simulink model "Y6MultirotorOpenLoopModelSimulation"  (R2019b)
settings: Solver=ode45  StartTime=0.0  StopTime=10  RelTol=1e-3  EnableMultiTasking=on
undefined symbols (not defined in the file or in its folder): Dxx, Dyy, Dzz, Ixx, Iyy, Izz, Ktau, Kthrust, Ku, Kw, L1, L2, L3, M, Mtau, U_e
settings Model: Creator=bjones  LastModifiedBy=alexd
settings DataIOCC: LimitDataPoints=on  SaveFormat=Array  SignalLoggingSaveFormat=ModelDataLogs  ReturnWorkspaceOutputs=off
settings OptimizationCC: ExpressionDepthLimit=2147483647  LifeSpan=inf
settings DebuggingCC: UnderspecifiedInitializationDetection=Classic  MergeDetectMultiDrivingBlocksExec=none  FcnCallInpInsideContextMsg=warning  StateNameClashWarn=warning  SFUnexpectedBacktrackingDiag=warning  SFNoUnconditionalDefaultTransitionDiag=warning  SFExecutionAtInitializationDiag=none  ArithmeticOperatorsInVariantConditions=warning
settings HardwareCC: ProdBitPerPointer=32  ProdBitPerSizeT=32  ProdBitPerPtrDiffT=32  ProdLargestAtomicFloat=None  ProdIntDivRoundTo=Undefined  ProdEndianess=Unspecified  ProdWordSize=32  ProdHWDeviceType=32-bit Generic
settings ModelReferenceCC: PropagateSignalLabelsOutOfModel=off
settings SFSimCC: SimUseLocalCustomCode=off  CustomCodeUndefinedFunction=UseInterfaceOnly
settings RTWCC: RTWUseLocalCustomCode=off
settings CodeAppCC: StateflowObjectComments=on
settings GRTTargetCC: TargetLangStandard=C89/C90 (ANSI)  GeneratePreprocessorConditionals=Disable all  CombineOutputUpdateFcns=off  GRTInterface=on
settings ConfigComp: CovMetricSettings=dw  CovHtmlReporting=on  CovSaveCumulativeToWorkspaceVar=on  CovSaveSingleToWorkspaceVar=on  CovExternalEMLEnable=off  CovSFcnEnable=off

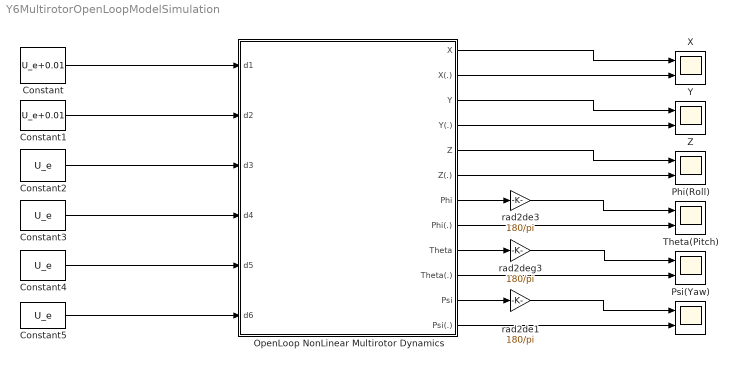
== system Y6MultirotorOpenLoopModelSimulation ==
  Constant : Constant  Value=U_e+0.01
  Constant1 : Constant  Value=U_e+0.01
  Constant{2..5} (4 alike) : Constant  Value=U_e
  OpenLoop NonLinear Multirotor Dynamics : Subsystem
  Phi(Roll) : Scope  NumInputPorts=2
  Psi(Yaw) : Scope  NumInputPorts=2
  Theta(Pitch) : Scope  NumInputPorts=2
  X : Scope  NumInputPorts=2
  Y : Scope  NumInputPorts=2
  Z : Scope  NumInputPorts=2
  rad2de1 : Gain  Gain=180/pi  SaturateOnIntegerOverflow=on  OutDataTypeStr=Inherit: Same as input  ParamDataTypeStr=Inherit: Same as input
  rad2de3 : Gain  Gain=180/pi  SaturateOnIntegerOverflow=on  OutDataTypeStr=Inherit: Same as input  ParamDataTypeStr=Inherit: Same as input
  rad2deg3 : Gain  Gain=180/pi  SaturateOnIntegerOverflow=on  OutDataTypeStr=Inherit: Same as input  ParamDataTypeStr=Inherit: Same as input
  wires:
  OpenLoop NonLinear Multirotor Dynamics/5(Z) -> Z/1
  OpenLoop NonLinear Multirotor Dynamics/1(X) -> X/1
  rad2deg3/1 -> Theta(Pitch)/1
  Constant/1 -> OpenLoop NonLinear Multirotor Dynamics/1(d1)
  Constant1/1 -> OpenLoop NonLinear Multirotor Dynamics/2(d2)
  OpenLoop NonLinear Multirotor Dynamics/3(Y) -> Y/1
  rad2de1/1 -> Psi(Yaw)/1
  rad2de3/1 -> Phi(Roll)/1
  Constant2/1 -> OpenLoop NonLinear Multirotor Dynamics/3(d3)
  Constant3/1 -> OpenLoop NonLinear Multirotor Dynamics/4(d4)
  Constant4/1 -> OpenLoop NonLinear Multirotor Dynamics/5(d5)
  Constant5/1 -> OpenLoop NonLinear Multirotor Dynamics/6(d6)
  OpenLoop NonLinear Multirotor Dynamics/7(Phi) -> rad2de3/1
  OpenLoop NonLinear Multirotor Dynamics/9(Theta) -> rad2deg3/1
  OpenLoop NonLinear Multirotor Dynamics/11(Psi) -> rad2de1/1
  OpenLoop NonLinear Multirotor Dynamics/12(Psi(.)) -> Psi(Yaw)/2
  OpenLoop NonLinear Multirotor Dynamics/10(Theta(.)) -> Theta(Pitch)/2
  OpenLoop NonLinear Multirotor Dynamics/8(Phi(.)) -> Phi(Roll)/2
  OpenLoop NonLinear Multirotor Dynamics/6(Z(.)) -> Z/2
  OpenLoop NonLinear Multirotor Dynamics/4(Y(.)) -> Y/2
  OpenLoop NonLinear Multirotor Dynamics/2(X(.)) -> X/2

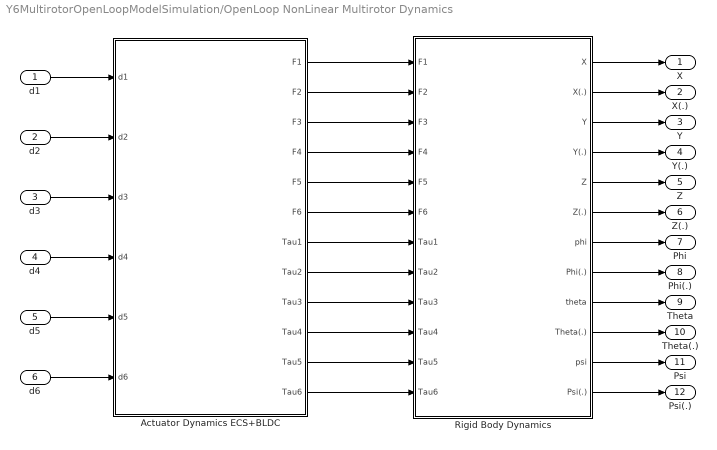
== system Y6MultirotorOpenLoopModelSimulation/OpenLoop NonLinear Multirotor Dynamics ==
  d1 : Inport
  d2 : Inport  Port=2
  d3 : Inport  Port=3
  d4 : Inport  Port=4
  d5 : Inport  Port=5
  d6 : Inport  Port=6
  Actuator Dynamics ECS+BLDC : Subsystem
  Rigid Body Dynamics : Subsystem
  X : Outport  VectorParamsAs1DForOutWhenUnconnected=off
  X(.) : Outport  Port=2  VectorParamsAs1DForOutWhenUnconnected=off
  Y : Outport  Port=3  VectorParamsAs1DForOutWhenUnconnected=off
  Y(.) : Outport  Port=4  VectorParamsAs1DForOutWhenUnconnected=off
  Z : Outport  Port=5  VectorParamsAs1DForOutWhenUnconnected=off
  Z(.) : Outport  Port=6  VectorParamsAs1DForOutWhenUnconnected=off
  Phi : Outport  Port=7  VectorParamsAs1DForOutWhenUnconnected=off
  Phi(.) : Outport  Port=8  VectorParamsAs1DForOutWhenUnconnected=off
  Theta : Outport  Port=9  VectorParamsAs1DForOutWhenUnconnected=off
  Theta(.) : Outport  Port=10  VectorParamsAs1DForOutWhenUnconnected=off
  Psi : Outport  Port=11  VectorParamsAs1DForOutWhenUnconnected=off
  Psi(.) : Outport  Port=12  VectorParamsAs1DForOutWhenUnconnected=off
  wires:
  Rigid Body Dynamics/7(phi) -> Phi/1
  Rigid Body Dynamics/8(Phi(.)) -> Phi(.)/1
  Rigid Body Dynamics/9(theta) -> Theta/1
  Rigid Body Dynamics/10(Theta(.)) -> Theta(.)/1
  Rigid Body Dynamics/11(psi) -> Psi/1
  Rigid Body Dynamics/12(Psi(.)) -> Psi(.)/1
  d1/1 -> Actuator Dynamics ECS+BLDC/1(d1)
  d2/1 -> Actuator Dynamics ECS+BLDC/2(d2)
  d3/1 -> Actuator Dynamics ECS+BLDC/3(d3)
  d4/1 -> Actuator Dynamics ECS+BLDC/4(d4)
  d5/1 -> Actuator Dynamics ECS+BLDC/5(d5)
  d6/1 -> Actuator Dynamics ECS+BLDC/6(d6)
  Actuator Dynamics ECS+BLDC/12(Tau6) -> Rigid Body Dynamics/12(Tau6)
  Actuator Dynamics ECS+BLDC/11(Tau5) -> Rigid Body Dynamics/11(Tau5)
  Actuator Dynamics ECS+BLDC/10(Tau4) -> Rigid Body Dynamics/10(Tau4)
  Actuator Dynamics ECS+BLDC/9(Tau3) -> Rigid Body Dynamics/9(Tau3)
  Actuator Dynamics ECS+BLDC/8(Tau2) -> Rigid Body Dynamics/8(Tau2)
  Actuator Dynamics ECS+BLDC/7(Tau1) -> Rigid Body Dynamics/7(Tau1)
  Actuator Dynamics ECS+BLDC/6(F6) -> Rigid Body Dynamics/6(F6)
  Actuator Dynamics ECS+BLDC/5(F5) -> Rigid Body Dynamics/5(F5)
  Actuator Dynamics ECS+BLDC/4(F4) -> Rigid Body Dynamics/4(F4)
  Actuator Dynamics ECS+BLDC/3(F3) -> Rigid Body Dynamics/3(F3)
  Actuator Dynamics ECS+BLDC/2(F2) -> Rigid Body Dynamics/2(F2)
  Actuator Dynamics ECS+BLDC/1(F1) -> Rigid Body Dynamics/1(F1)
  Rigid Body Dynamics/6(Z(.)) -> Z(.)/1
  Rigid Body Dynamics/5(Z) -> Z/1
  Rigid Body Dynamics/4(Y(.)) -> Y(.)/1
  Rigid Body Dynamics/3(Y) -> Y/1
  Rigid Body Dynamics/2(X(.)) -> X(.)/1
  Rigid Body Dynamics/1(X) -> X/1

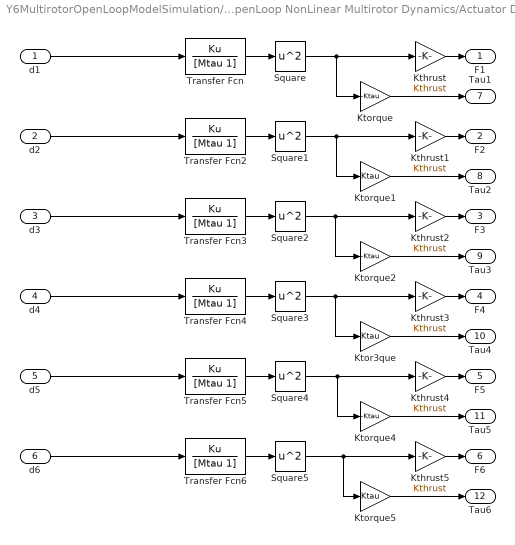
== system Y6MultirotorOpenLoopModelSimulation/OpenLoop NonLinear Multirotor Dynamics/Actuator Dynamics ECS+BLDC ==
  d1 : Inport
  d2 : Inport  Port=2
  d3 : Inport  Port=3
  d4 : Inport  Port=4
  d5 : Inport  Port=5
  d6 : Inport  Port=6
  Kthrust{,1..5} (6 alike) : Gain  Gain=Kthrust
  Ktor3que : Gain  Gain=Ktau
  Ktorque : Gain  Gain=-Ktau
  Ktorque1 : Gain  Gain=Ktau
  Ktorque2 : Gain  Gain=-Ktau
  Ktorque4 : Gain  Gain=-Ktau
  Ktorque5 : Gain  Gain=Ktau
  Square{,1..5} (6 alike) : Math  Operator=square  SignedPower=off  SaturateOnIntegerOverflow=on
  Transfer Fcn{,2..6} (6 alike) : TransferFcn  Numerator=Ku  Denominator=[Mtau 1]
  F1 : Outport  VectorParamsAs1DForOutWhenUnconnected=off
  F2 : Outport  Port=2  VectorParamsAs1DForOutWhenUnconnected=off
  F3 : Outport  Port=3  VectorParamsAs1DForOutWhenUnconnected=off
  F4 : Outport  Port=4  VectorParamsAs1DForOutWhenUnconnected=off
  F5 : Outport  Port=5  VectorParamsAs1DForOutWhenUnconnected=off
  F6 : Outport  Port=6  VectorParamsAs1DForOutWhenUnconnected=off
  Tau1 : Outport  Port=7  VectorParamsAs1DForOutWhenUnconnected=off
  Tau2 : Outport  Port=8  VectorParamsAs1DForOutWhenUnconnected=off
  Tau3 : Outport  Port=9  VectorParamsAs1DForOutWhenUnconnected=off
  Tau4 : Outport  Port=10  VectorParamsAs1DForOutWhenUnconnected=off
  Tau5 : Outport  Port=11  VectorParamsAs1DForOutWhenUnconnected=off
  Tau6 : Outport  Port=12  VectorParamsAs1DForOutWhenUnconnected=off
  wires:
  Transfer Fcn/1 -> Square/1
  d1/1 -> Transfer Fcn/1
  d2/1 -> Transfer Fcn2/1
  d3/1 -> Transfer Fcn3/1
  d4/1 -> Transfer Fcn4/1
  d5/1 -> Transfer Fcn5/1
  d6/1 -> Transfer Fcn6/1
  Transfer Fcn2/1 -> Square1/1
  Transfer Fcn3/1 -> Square2/1
  Transfer Fcn4/1 -> Square3/1
  Transfer Fcn5/1 -> Square4/1
  Transfer Fcn6/1 -> Square5/1
  Ktorque/1 -> Tau1/1
  Ktorque1/1 -> Tau2/1
  Ktorque2/1 -> Tau3/1
  Ktor3que/1 -> Tau4/1
  Ktorque4/1 -> Tau5/1
  Ktorque5/1 -> Tau6/1
  Kthrust/1 -> F1/1
  Kthrust1/1 -> F2/1
  Kthrust2/1 -> F3/1
  Kthrust3/1 -> F4/1
  Kthrust4/1 -> F5/1
  Kthrust5/1 -> F6/1
  Square/1 -> Kthrust/1, Ktorque/1
  Square1/1 -> Kthrust1/1, Ktorque1/1
  Square2/1 -> Kthrust2/1, Ktorque2/1
  Square3/1 -> Kthrust3/1, Ktor3que/1
  Square4/1 -> Kthrust4/1, Ktorque4/1
  Square5/1 -> Kthrust5/1, Ktorque5/1

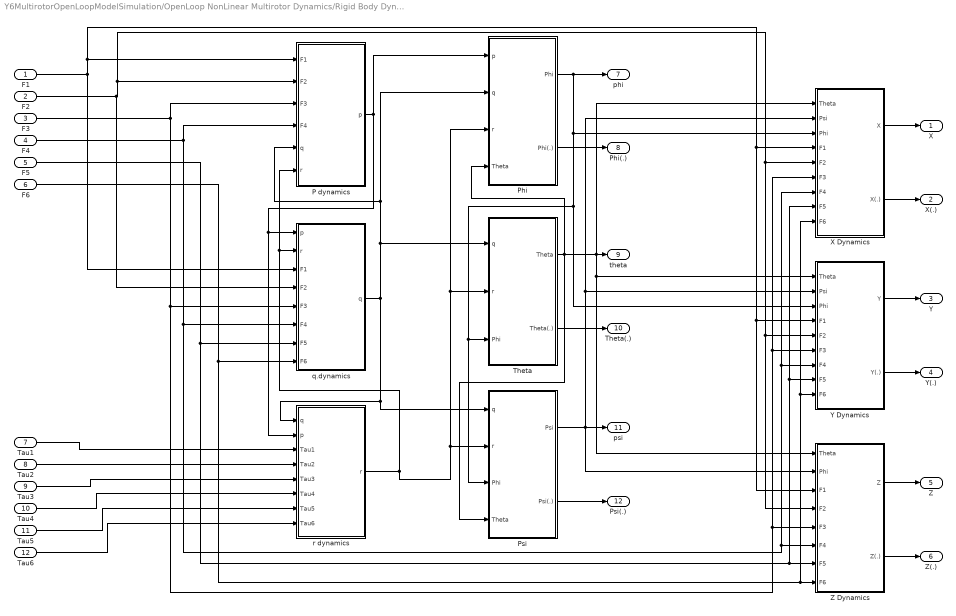
== system Y6MultirotorOpenLoopModelSimulation/OpenLoop NonLinear Multirotor Dynamics/Rigid Body Dynamics ==
  F1 : Inport
  F2 : Inport  Port=2
  F3 : Inport  Port=3
  F4 : Inport  Port=4
  F5 : Inport  Port=5
  F6 : Inport  Port=6
  Tau1 : Inport  Port=7
  Tau2 : Inport  Port=8
  Tau3 : Inport  Port=9
  Tau4 : Inport  Port=10
  Tau5 : Inport  Port=11
  Tau6 : Inport  Port=12
  P dynamics : Subsystem
  Phi : Subsystem
  Psi : Subsystem
  Theta : Subsystem
  X Dynamics : Subsystem
  Y Dynamics : Subsystem
  Z Dynamics : Subsystem
  q.dynamics : Subsystem
  r dynamics : Subsystem
  X : Outport  VectorParamsAs1DForOutWhenUnconnected=off
  X(.) : Outport  Port=2  VectorParamsAs1DForOutWhenUnconnected=off
  Y : Outport  Port=3  VectorParamsAs1DForOutWhenUnconnected=off
  Y(.) : Outport  Port=4  VectorParamsAs1DForOutWhenUnconnected=off
  Z : Outport  Port=5  VectorParamsAs1DForOutWhenUnconnected=off
  Z(.) : Outport  Port=6  VectorParamsAs1DForOutWhenUnconnected=off
  phi : Outport  Port=7  VectorParamsAs1DForOutWhenUnconnected=off
  Phi(.) : Outport  Port=8  VectorParamsAs1DForOutWhenUnconnected=off
  theta : Outport  Port=9  VectorParamsAs1DForOutWhenUnconnected=off
  Theta(.) : Outport  Port=10  VectorParamsAs1DForOutWhenUnconnected=off
  psi : Outport  Port=11  VectorParamsAs1DForOutWhenUnconnected=off
  Psi(.) : Outport  Port=12  VectorParamsAs1DForOutWhenUnconnected=off
  wires:
  Tau2/1 -> r dynamics/4(Tau2)
  Tau3/1 -> r dynamics/5(Tau3)
  Tau4/1 -> r dynamics/6(Tau4)
  Tau5/1 -> r dynamics/7(Tau5)
  Tau6/1 -> r dynamics/8(Tau6)
  F2/1 -> q.dynamics/4("F2 "), X Dynamics/5("F2 "), Z Dynamics/4("F2 "), Y Dynamics/5("F2 "), P dynamics/2(F2)
  F3/1 -> q.dynamics/5("F3 "), X Dynamics/6("F3 "), Y Dynamics/6("F3 "), Z Dynamics/5("F3 "), P dynamics/3(F3)
  F4/1 -> P dynamics/4(F4), q.dynamics/6("F4 "), X Dynamics/7("F4 "), Y Dynamics/7("F4 "), Z Dynamics/6("F4 ")
  Tau1/1 -> r dynamics/3(Tau1)
  r dynamics/1(r) -> Phi/3(r), Theta/2(r), Psi/2(r), P dynamics/6(r), q.dynamics/2(r)
  F1/1 -> Z Dynamics/3("F1 "), Y Dynamics/4("F1 "), X Dynamics/4("F1 "), P dynamics/1(F1), q.dynamics/3("F1 ")
  F5/1 -> q.dynamics/7("F5 "), Y Dynamics/8("F5 "), X Dynamics/8("F5 "), Z Dynamics/7("F5 ")
  F6/1 -> Y Dynamics/9(F6), X Dynamics/9(F6), Z Dynamics/8(F6), q.dynamics/8(F6)
  Z Dynamics/1(Z) -> Z/1
  Z Dynamics/2(Z(.)) -> Z(.)/1
  Y Dynamics/2(Y(.)) -> Y(.)/1
  Y Dynamics/1(Y) -> Y/1
  X Dynamics/2(X(.)) -> X(.)/1
  X Dynamics/1(X) -> X/1
  Phi/1(Phi) -> phi/1, X Dynamics/3(Phi), Y Dynamics/3(Phi), Theta/3(Phi), Psi/3(Phi)
  Theta/1(Theta) -> X Dynamics/1(Theta), theta/1, Y Dynamics/1(Theta), Z Dynamics/1(Theta), Phi/4(Theta), Psi/4(Theta)
  Theta/2(Theta(.)) -> Theta(.)/1
  Phi/2(Phi(.)) -> Phi(.)/1
  Psi/1(Psi) -> Z Dynamics/2(Phi), psi/1, X Dynamics/2(Psi), Y Dynamics/2(Psi)
  Psi/2(Psi(.)) -> Psi(.)/1
  q.dynamics/1(q) -> r dynamics/1(q), Psi/1(q), Theta/1(q), Phi/2(q), P dynamics/5(q)
  P dynamics/1(p) -> Phi/1(p), q.dynamics/1(p), r dynamics/2(p)

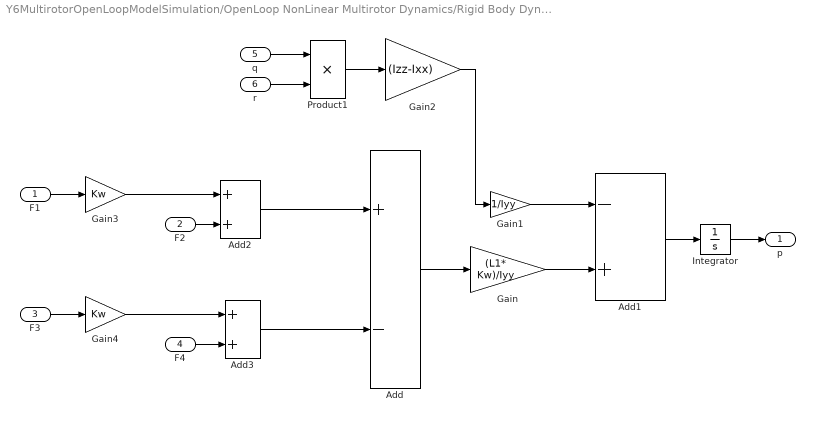
== system Y6MultirotorOpenLoopModelSimulation/OpenLoop NonLinear Multirotor Dynamics/Rigid Body Dynamics/P dynamics ==
  F1 : Inport
  F2 : Inport  Port=2
  F3 : Inport  Port=3
  F4 : Inport  Port=4
  q : Inport  Port=5
  r : Inport  Port=6
  Add : Sum  Inputs=+-
  Add1 : Sum  Inputs=-+
  Add2 : Sum
  Add3 : Sum
  Gain : Gain  Gain=(L1* Kw)/Iyy
  Gain1 : Gain  Gain=1/Iyy
  Gain2 : Gain  Gain=(Izz-Ixx)
  Gain3 : Gain  Gain=Kw
  Gain4 : Gain  Gain=Kw
  Integrator : Integrator
  Product1 : Product
  p : Outport  VectorParamsAs1DForOutWhenUnconnected=off
  wires:
  Product1/1 -> Gain2/1
  Add1/1 -> Integrator/1
  Gain1/1 -> Add1/1
  Add/1 -> Gain/1
  Gain2/1 -> Gain1/1
  Gain/1 -> Add1/2
  F4/1 -> Add3/2
  F3/1 -> Gain4/1
  Add2/1 -> Add/1
  Add3/1 -> Add/2
  Integrator/1 -> p/1
  r/1 -> Product1/2
  q/1 -> Product1/1
  F2/1 -> Add2/2
  F1/1 -> Gain3/1
  Gain3/1 -> Add2/1
  Gain4/1 -> Add3/1

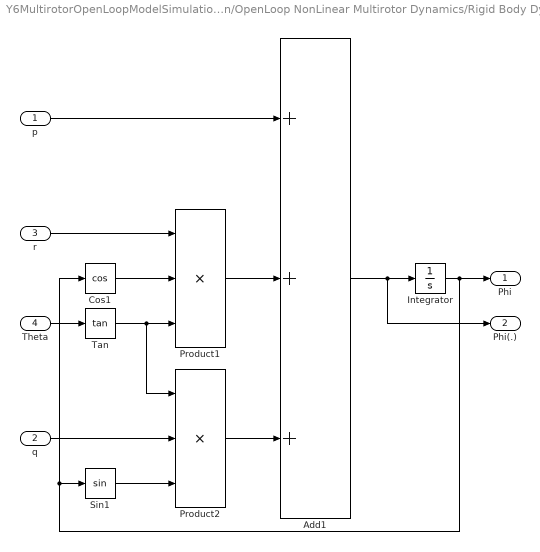
== system Y6MultirotorOpenLoopModelSimulation/OpenLoop NonLinear Multirotor Dynamics/Rigid Body Dynamics/Phi ==
  p : Inport
  q : Inport  Port=2
  r : Inport  Port=3
  Theta : Inport  Port=4
  Add1 : Sum  Inputs=+++
  Cos1 : Trigonometry  Operator=cos
  Integrator : Integrator
  Product1 : Product  Inputs=3
  Product2 : Product  Inputs=3
  Sin1 : Trigonometry
  Tan : Trigonometry  Operator=tan
  Phi : Outport  VectorParamsAs1DForOutWhenUnconnected=off
  Phi(.) : Outport  Port=2  VectorParamsAs1DForOutWhenUnconnected=off
  wires:
  p/1 -> Add1/1
  Theta/1 -> Tan/1
  Tan/1 -> Product2/1, Product1/3
  r/1 -> Product1/1
  Cos1/1 -> Product1/2
  Sin1/1 -> Product2/3
  q/1 -> Product2/2
  Product1/1 -> Add1/2
  Product2/1 -> Add1/3
  Add1/1 -> Phi(.)/1, Integrator/1
  Integrator/1 -> Cos1/1, Sin1/1, Phi/1

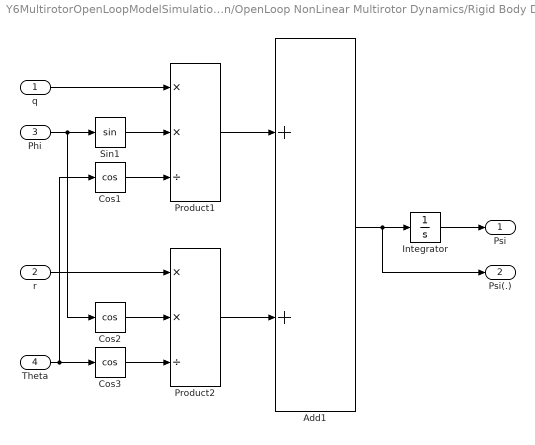
== system Y6MultirotorOpenLoopModelSimulation/OpenLoop NonLinear Multirotor Dynamics/Rigid Body Dynamics/Psi ==
  q : Inport
  r : Inport  Port=2
  Phi : Inport  Port=3
  Theta : Inport  Port=4
  Add1 : Sum
  Cos1 : Trigonometry  Operator=cos
  Cos2 : Trigonometry  Operator=cos
  Cos3 : Trigonometry  Operator=cos
  Integrator : Integrator
  Product1 : Product  Inputs=**/
  Product2 : Product  Inputs=**/
  Sin1 : Trigonometry
  Psi : Outport  VectorParamsAs1DForOutWhenUnconnected=off
  Psi(.) : Outport  Port=2  VectorParamsAs1DForOutWhenUnconnected=off
  wires:
  Add1/1 -> Integrator/1, Psi(.)/1
  Integrator/1 -> Psi/1
  Product1/1 -> Add1/1
  Product2/1 -> Add1/2
  Phi/1 -> Sin1/1, Cos2/1
  r/1 -> Product2/1
  q/1 -> Product1/1
  Cos2/1 -> Product2/2
  Cos3/1 -> Product2/3
  Theta/1 -> Cos1/1, Cos3/1
  Cos1/1 -> Product1/3
  Sin1/1 -> Product1/2

== system Y6MultirotorOpenLoopModelSimulation/OpenLoop NonLinear Multirotor Dynamics/Rigid Body Dynamics/Theta ==
  q : Inport
  r : Inport  Port=2
  Phi : Inport  Port=3
  Add1 : Sum  Inputs=+-
  Cos1 : Trigonometry  Operator=cos
  Integrator : Integrator
  Product1 : Product
  Product2 : Product
  Sin1 : Trigonometry
  Theta : Outport  VectorParamsAs1DForOutWhenUnconnected=off
  Theta(.) : Outport  Port=2  VectorParamsAs1DForOutWhenUnconnected=off
  wires:
  Cos1/1 -> Product1/2
  Add1/1 -> Integrator/1, Theta(.)/1
  Integrator/1 -> Theta/1
  Product1/1 -> Add1/1
  Product2/1 -> Add1/2
  Phi/1 -> Sin1/1, Cos1/1
  Sin1/1 -> Product2/2
  r/1 -> Product2/1
  q/1 -> Product1/1

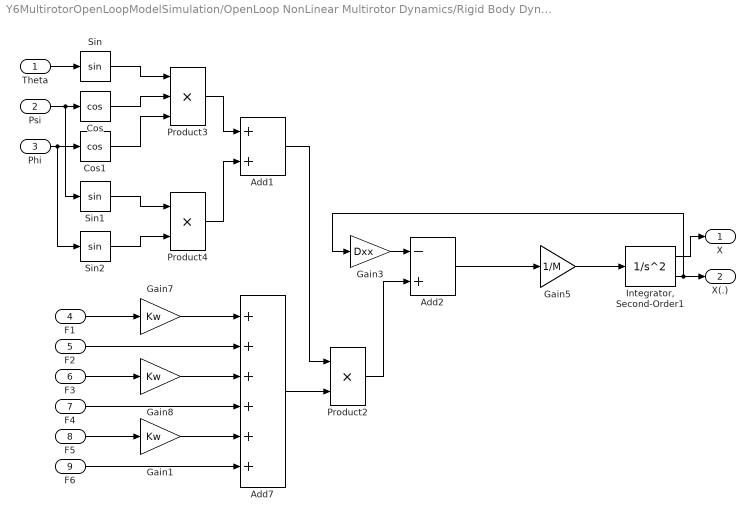
== system Y6MultirotorOpenLoopModelSimulation/OpenLoop NonLinear Multirotor Dynamics/Rigid Body Dynamics/X Dynamics ==
  Theta : Inport
  Psi : Inport  Port=2
  Phi : Inport  Port=3
  "F1 " : Inport  Port=4
  "F2 " : Inport  Port=5
  "F3 " : Inport  Port=6
  "F4 " : Inport  Port=7
  "F5 " : Inport  Port=8
  F6 : Inport  Port=9
  Add1 : Sum
  Add2 : Sum  Inputs=-+
  Add7 : Sum  Inputs=++++++
  Cos : Trigonometry  Operator=cos
  Cos1 : Trigonometry  Operator=cos
  Gain1 : Gain  Gain=Kw
  Gain3 : Gain  Gain=Dxx
  Gain5 : Gain  Gain=1/M
  Gain7 : Gain  Gain=Kw
  Gain8 : Gain  Gain=Kw
  "Integrator, Second-Order1" : SecondOrderIntegrator
  Product2 : Product
  Product3 : Product  Inputs=3
  Product4 : Product
  Sin : Trigonometry
  Sin1 : Trigonometry
  Sin2 : Trigonometry
  X : Outport  VectorParamsAs1DForOutWhenUnconnected=off
  X(.) : Outport  Port=2  VectorParamsAs1DForOutWhenUnconnected=off
  wires:
  "F4 "/1 -> Add7/4
  "F2 "/1 -> Add7/2
  "Integrator, Second-Order1"/2 -> X(.)/1, Gain3/1
  "F1 "/1 -> Gain7/1
  F6/1 -> Add7/6
  "F5 "/1 -> Gain1/1
  "F3 "/1 -> Gain8/1
  "Integrator, Second-Order1"/1 -> X/1
  Gain7/1 -> Add7/1
  Gain8/1 -> Add7/3
  Gain1/1 -> Add7/5
  Add7/1 -> Product2/2
  Theta/1 -> Sin/1
  Psi/1 -> Sin1/1, Cos/1
  Phi/1 -> Sin2/1, Cos1/1
  Sin/1 -> Product3/1
  Cos/1 -> Product3/2
  Cos1/1 -> Product3/3
  Product3/1 -> Add1/1
  Sin1/1 -> Product4/1
  Sin2/1 -> Product4/2
  Product4/1 -> Add1/2
  Add1/1 -> Product2/1
  Product2/1 -> Add2/2
  Add2/1 -> Gain5/1
  Gain3/1 -> Add2/1
  Gain5/1 -> "Integrator, Second-Order1"/1

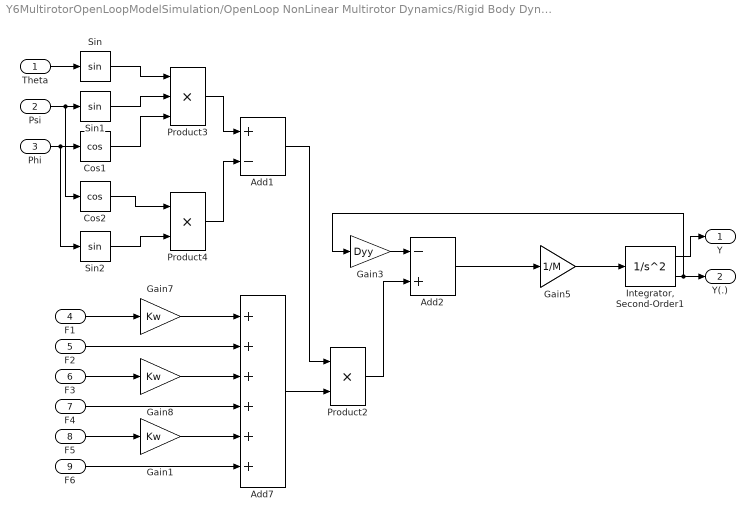
== system Y6MultirotorOpenLoopModelSimulation/OpenLoop NonLinear Multirotor Dynamics/Rigid Body Dynamics/Y Dynamics ==
  Theta : Inport
  Psi : Inport  Port=2
  Phi : Inport  Port=3
  "F1 " : Inport  Port=4
  "F2 " : Inport  Port=5
  "F3 " : Inport  Port=6
  "F4 " : Inport  Port=7
  "F5 " : Inport  Port=8
  F6 : Inport  Port=9
  Add1 : Sum  Inputs=+-
  Add2 : Sum  Inputs=-+
  Add7 : Sum  Inputs=++++++
  Cos1 : Trigonometry  Operator=cos
  Cos2 : Trigonometry  Operator=cos
  Gain1 : Gain  Gain=Kw
  Gain3 : Gain  Gain=Dyy
  Gain5 : Gain  Gain=1/M
  Gain7 : Gain  Gain=Kw
  Gain8 : Gain  Gain=Kw
  "Integrator, Second-Order1" : SecondOrderIntegrator
  Product2 : Product
  Product3 : Product  Inputs=3
  Product4 : Product
  Sin : Trigonometry
  Sin1 : Trigonometry
  Sin2 : Trigonometry
  Y : Outport  VectorParamsAs1DForOutWhenUnconnected=off
  Y(.) : Outport  Port=2  VectorParamsAs1DForOutWhenUnconnected=off
  wires:
  "F4 "/1 -> Add7/4
  "F2 "/1 -> Add7/2
  "Integrator, Second-Order1"/2 -> Y(.)/1, Gain3/1
  "F1 "/1 -> Gain7/1
  F6/1 -> Add7/6
  "F5 "/1 -> Gain1/1
  "F3 "/1 -> Gain8/1
  "Integrator, Second-Order1"/1 -> Y/1
  Gain7/1 -> Add7/1
  Gain8/1 -> Add7/3
  Gain1/1 -> Add7/5
  Add7/1 -> Product2/2
  Theta/1 -> Sin/1
  Phi/1 -> Sin2/1, Cos1/1
  Sin/1 -> Product3/1
  Psi/1 -> Sin1/1, Cos2/1
  Cos1/1 -> Product3/3
  Product3/1 -> Add1/1
  Sin2/1 -> Product4/2
  Product4/1 -> Add1/2
  Add1/1 -> Product2/1
  Product2/1 -> Add2/2
  Add2/1 -> Gain5/1
  Gain3/1 -> Add2/1
  Gain5/1 -> "Integrator, Second-Order1"/1
  Cos2/1 -> Product4/1
  Sin1/1 -> Product3/2

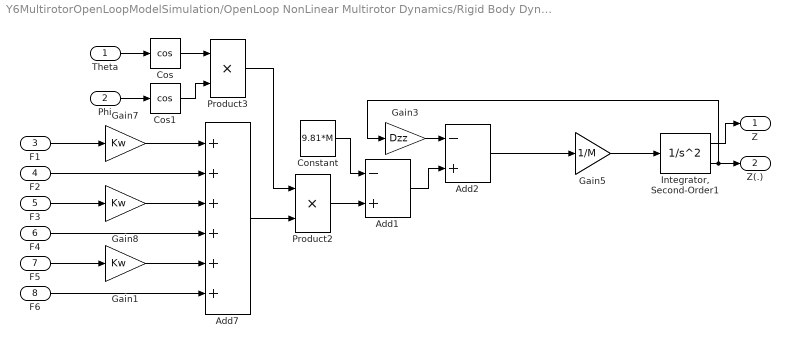
== system Y6MultirotorOpenLoopModelSimulation/OpenLoop NonLinear Multirotor Dynamics/Rigid Body Dynamics/Z Dynamics ==
  Theta : Inport
  Phi : Inport  Port=2
  "F1 " : Inport  Port=3
  "F2 " : Inport  Port=4
  "F3 " : Inport  Port=5
  "F4 " : Inport  Port=6
  "F5 " : Inport  Port=7
  F6 : Inport  Port=8
  Add1 : Sum  Inputs=-+
  Add2 : Sum  Inputs=-+
  Add7 : Sum  Inputs=++++++
  Constant : Constant  Value=9.81*M
  Cos : Trigonometry  Operator=cos
  Cos1 : Trigonometry  Operator=cos
  Gain1 : Gain  Gain=Kw
  Gain3 : Gain  Gain=Dzz
  Gain5 : Gain  Gain=1/M
  Gain7 : Gain  Gain=Kw
  Gain8 : Gain  Gain=Kw
  "Integrator, Second-Order1" : SecondOrderIntegrator
  Product2 : Product
  Product3 : Product
  Z : Outport  VectorParamsAs1DForOutWhenUnconnected=off
  Z(.) : Outport  Port=2  VectorParamsAs1DForOutWhenUnconnected=off
  wires:
  "F4 "/1 -> Add7/4
  "F2 "/1 -> Add7/2
  "Integrator, Second-Order1"/2 -> Z(.)/1, Gain3/1
  "F1 "/1 -> Gain7/1
  F6/1 -> Add7/6
  "F5 "/1 -> Gain1/1
  "F3 "/1 -> Gain8/1
  "Integrator, Second-Order1"/1 -> Z/1
  Gain7/1 -> Add7/1
  Gain8/1 -> Add7/3
  Gain1/1 -> Add7/5
  Add7/1 -> Product2/2
  Theta/1 -> Cos/1
  Phi/1 -> Cos1/1
  Product3/1 -> Product2/1
  Add2/1 -> Gain5/1
  Gain3/1 -> Add2/1
  Gain5/1 -> "Integrator, Second-Order1"/1
  Cos/1 -> Product3/1
  Cos1/1 -> Product3/2
  Product2/1 -> Add1/2
  Add1/1 -> Add2/2
  Constant/1 -> Add1/1

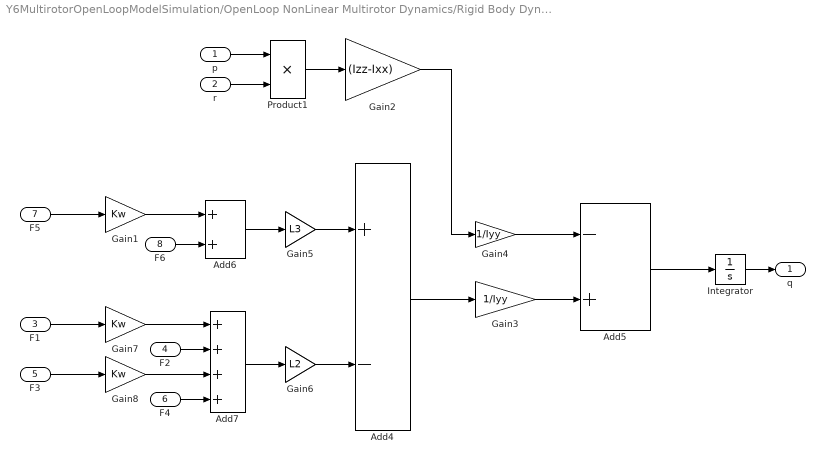
== system Y6MultirotorOpenLoopModelSimulation/OpenLoop NonLinear Multirotor Dynamics/Rigid Body Dynamics/q.dynamics ==
  p : Inport
  r : Inport  Port=2
  "F1 " : Inport  Port=3
  "F2 " : Inport  Port=4
  "F3 " : Inport  Port=5
  "F4 " : Inport  Port=6
  "F5 " : Inport  Port=7
  F6 : Inport  Port=8
  Add4 : Sum  Inputs=+-
  Add5 : Sum  Inputs=-+
  Add6 : Sum
  Add7 : Sum  Inputs=++++
  Gain1 : Gain  Gain=Kw
  Gain2 : Gain  Gain=(Izz-Ixx)
  Gain3 : Gain  Gain=1/Iyy
  Gain4 : Gain  Gain=1/Iyy
  Gain5 : Gain  Gain=L3
  Gain6 : Gain  Gain=L2
  Gain7 : Gain  Gain=Kw
  Gain8 : Gain  Gain=Kw
  Integrator : Integrator
  Product1 : Product
  q : Outport  VectorParamsAs1DForOutWhenUnconnected=off
  wires:
  p/1 -> Product1/1
  r/1 -> Product1/2
  Product1/1 -> Gain2/1
  "F4 "/1 -> Add7/4
  Gain5/1 -> Add4/1
  "F2 "/1 -> Add7/2
  Add7/1 -> Gain6/1
  "F1 "/1 -> Gain7/1
  Gain3/1 -> Add5/2
  F6/1 -> Add6/2
  "F5 "/1 -> Gain1/1
  Add6/1 -> Gain5/1
  "F3 "/1 -> Gain8/1
  Gain6/1 -> Add4/2
  Gain4/1 -> Add5/1
  Gain2/1 -> Gain4/1
  Add4/1 -> Gain3/1
  Add5/1 -> Integrator/1
  Gain1/1 -> Add6/1
  Gain7/1 -> Add7/1
  Gain8/1 -> Add7/3
  Integrator/1 -> q/1

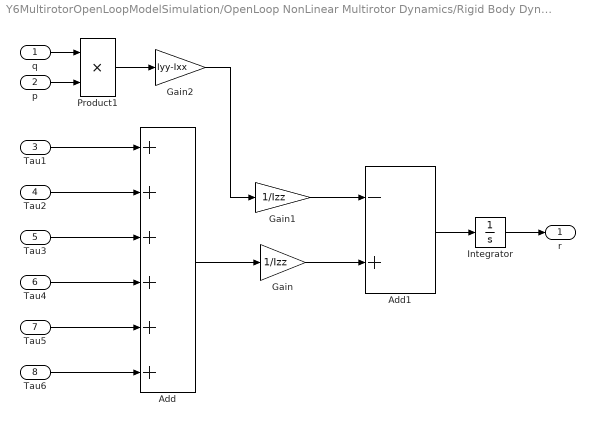
== system Y6MultirotorOpenLoopModelSimulation/OpenLoop NonLinear Multirotor Dynamics/Rigid Body Dynamics/r dynamics ==
  q : Inport
  p : Inport  Port=2
  Tau1 : Inport  Port=3
  Tau2 : Inport  Port=4
  Tau3 : Inport  Port=5
  Tau4 : Inport  Port=6
  Tau5 : Inport  Port=7
  Tau6 : Inport  Port=8
  Add : Sum  Inputs=++++++
  Add1 : Sum  Inputs=-+
  Gain : Gain  Gain=1/Izz
  Gain1 : Gain  Gain=1/Izz
  Gain2 : Gain  Gain=Iyy-Ixx
  Integrator : Integrator
  Product1 : Product
  r : Outport  VectorParamsAs1DForOutWhenUnconnected=off
  wires:
  Tau6/1 -> Add/6
  Tau5/1 -> Add/5
  Tau4/1 -> Add/4
  Tau3/1 -> Add/3
  Tau2/1 -> Add/2
  Tau1/1 -> Add/1
  Add/1 -> Gain/1
  Gain/1 -> Add1/2
  Gain1/1 -> Add1/1
  Gain2/1 -> Gain1/1
  q/1 -> Product1/1
  p/1 -> Product1/2
  Product1/1 -> Gain2/1
  Add1/1 -> Integrator/1
  Integrator/1 -> r/1
